simulink model "adc_ut"  (Simulink 8.1)
settings: Solver=FixedStepDiscrete  StartTime=0.0  StopTime=Inf  FixedStep=0.005  RelTol=1e-3
PostLoadFcn:
  | , if any(exist('dsrtsu_mdlpostloadfcn', 'file') == [2, 3, 6]), try dsrtsu_mdlpostloadfcn('Execute', bdroot); catch fprintf('Error in PostLoadFcn (dsrtsu_mdlpostloadfcn) for model "%s":\n %s\n', bdroot, lasterr); end, end,
libraries: adc x1
settings Model: DSRTSU_INTERNAL_RTI_VER=450  DSRTSU_INTERNAL_RTI_TYPE=rti1401  RTICANMMDATA=struct('GeneralSetupData',struct('modelroot','D:\ELN150201_TAIWAN\trunk\AdasDragon\software\sw_development\arch\app\jud','generalsettings',struct('filesettings',struct('destfolder',struct('Name','RTICANMM_FILES','Check',1),'buildfolder',struct('Name','.','Check',1),'AbsDestfolder',struct('Name','D:\ELN150201_TAIWAN\trunk\AdasDragon\software\sw_development\arch\app\jud\RTICANMM_FILES'),'AbsBuildfolder',struct('Name','D:\ELN150201_TAIWAN\trunk\AdasDragon\software\sw_development\arch\app\jud'))),'options',struct('addpaths',1,'rmpaths',1,'addtrcexclusion',logical(1),'cannavigator',struct('checkmonitoring',0),'show_usrtrc',0,'use_usrtrc',0),'advanced',struct('options',[1 1 1 1 1 1 1 1 1 1 1 1 1 1 1 1 1 1 1 1 1 1 1 1 1 1 1 1 1 1 1 1 1 1 1 1 1 1 1 1 1 1 1 1 1 1 1 1 1 1 1 1 1 1 1 1 1 1 1 1 1 1 1 1 1 1 1 1 1 1 1 1 1 1 1 1 1 1 1 1 1 1 1 1 1 1 1 1 1 1 1 1 1 1 1 1 1 1 1 1]),'MPSetup',{{}},'modelname','adc_ut','block','adc_ut'))  DSRTSU_INTERNAL_RTIFPGA=40  Creator=AT015411  LastModifiedBy=AT015555  BufferReuse=off
settings DataIOCC: SignalLoggingSaveFormat=Dataset
settings OptimizationCC: BlockReduction=off  OptimizeBlockIOStorage=off  BufferReuse=off  ExpressionFolding=off  ExpressionDepthLimit=128  LocalBlockOutputs=off
settings DebuggingCC: FcnCallInpInsideContextMsg=EnableAllAsError
settings HardwareCC: ProdIntDivRoundTo=Zero  ProdEndianess=BigEndian  ProdHWDeviceType=Generic->Custom  TargetIntDivRoundTo=Zero  TargetEndianess=BigEndian  TargetHWDeviceType=Generic->Custom
settings RTWCC: SystemTargetFile=rti1005.tlc  MakeCommand=make_rti  TemplateMakefile=rti1005.tmf  Description=dSPACE DS1005 Hardware Platform  ProcessScript=rti1005_make_rtw_hook
settings STFCustomTargetCC: CodeReplacementLibrary=ANSI_C  ParMdlRefBuildCompliant=on  GeneratePreprocessorConditionals=Disable all  MatFileLogging=on  SystemTargetFile=rti1005.tlc
settings GRTTargetCC: CompOptLevelCompliant=off  ConcurrentExecutionCompliant=off  ExtModeMexFile=noextcomm
settings CustomProperty: DataType=RTWOptions_EnumType_C__Program Files (x86)_dSPACE RCPHIL 2014-B_MATLAB_RTI_RTI1401_TLC_rti1005_1InitialSimState  Value=RUN
settings EnumStrPairs: String=RUN

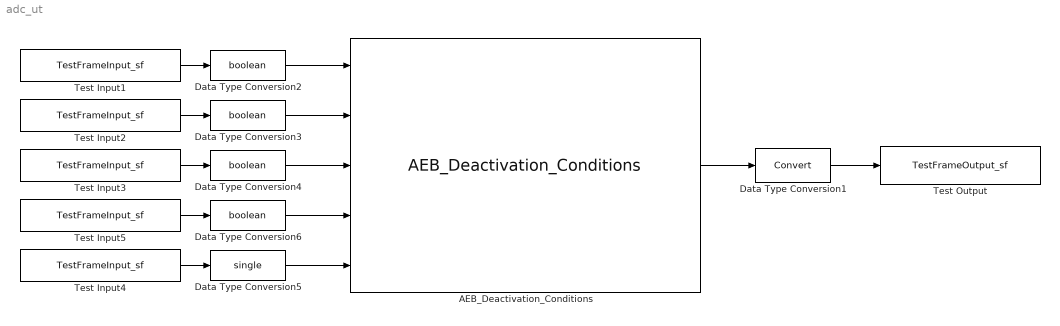
== system adc_ut ==
  AEB_Deactivation_Conditions : adc/AEB_Deactivation_Conditions
  Data Type Conversion1 : DataTypeConversion
  Data Type Conversion{2..4,6} (4 alike) : DataTypeConversion  OutDataTypeStr=boolean
  Data Type Conversion5 : DataTypeConversion  OutDataTypeStr=single
  Test Input1 : S-Function  FunctionName=TestFrameInput_sf  Parameters=varname,sampletime  EnableBusSupport=off  mask(Test Input){varname=VIFO_ParkingSituation_flg, sampletime=0.005}
      mask prompts: varname "Name:"; sampletime "Sample Time:"
      mask help: Outputs the value of a Test Input variable from an Excel spreadsheet when used with the runsiltest script. Otherwise outputs 0.
      mask Display: fprintf('Test Input:\n%s',varname);
  Test Input2 : S-Function  FunctionName=TestFrameInput_sf  Parameters=varname,sampletime  EnableBusSupport=off  mask(Test Input){varname=VIFO_DriverOverrideReq_flg, sampletime=0.005}
      mask prompts: varname "Name:"; sampletime "Sample Time:"
      mask help: Outputs the value of a Test Input variable from an Excel spreadsheet when used with the runsiltest script. Otherwise outputs 0.
      mask Display: fprintf('Test Input:\n%s',varname);
  Test Input3 : S-Function  FunctionName=TestFrameInput_sf  Parameters=varname,sampletime  EnableBusSupport=off  mask(Test Input){varname=VIFO_AEBTargetVehAssigned_flg, sampletime=0.005}
      mask prompts: varname "Name:"; sampletime "Sample Time:"
      mask help: Outputs the value of a Test Input variable from an Excel spreadsheet when used with the runsiltest script. Otherwise outputs 0.
      mask Display: fprintf('Test Input:\n%s',varname);
  Test Input4 : S-Function  FunctionName=TestFrameInput_sf  Parameters=varname,sampletime  EnableBusSupport=off  mask(Test Input){varname=VDINR_VehSpd_mps, sampletime=0.005}
      mask prompts: varname "Name:"; sampletime "Sample Time:"
      mask help: Outputs the value of a Test Input variable from an Excel spreadsheet when used with the runsiltest script. Otherwise outputs 0.
      mask Display: fprintf('Test Input:\n%s',varname);
  Test Input5 : S-Function  FunctionName=TestFrameInput_sf  Parameters=varname,sampletime  EnableBusSupport=off  mask(Test Input){varname=VIFO_VRUTargetPedAssigned_flg, sampletime=0.005}
      mask prompts: varname "Name:"; sampletime "Sample Time:"
      mask help: Outputs the value of a Test Input variable from an Excel spreadsheet when used with the runsiltest script. Otherwise outputs 0.
      mask Display: fprintf('Test Input:\n%s',varname);
  Test Output : S-Function  FunctionName=TestFrameOutput_sf  Parameters=varname,sampletime  EnableBusSupport=off  mask(Test Output){varname=VJUD_AEBDeactivationReq_flg, sampletime=-1}
      mask prompts: varname "Name:"; sampletime "Sample Time:"
      mask help: Samples the value of a Test Output variable from an Excel spreadsheet when used with the runsiltest script. Otherwise does nothing.
      mask Display: fprintf('Test Output:\n%s',varname);
  wires:
  AEB_Deactivation_Conditions/1 -> Data Type Conversion1/1
  Data Type Conversion1/1 -> Test Output/1
  Test Input1/1 -> Data Type Conversion2/1
  Data Type Conversion2/1 -> AEB_Deactivation_Conditions/1
  Test Input2/1 -> Data Type Conversion3/1
  Data Type Conversion3/1 -> AEB_Deactivation_Conditions/2
  Test Input3/1 -> Data Type Conversion4/1
  Data Type Conversion4/1 -> AEB_Deactivation_Conditions/3
  Test Input4/1 -> Data Type Conversion5/1
  Data Type Conversion5/1 -> AEB_Deactivation_Conditions/5
  Test Input5/1 -> Data Type Conversion6/1
  Data Type Conversion6/1 -> AEB_Deactivation_Conditions/4
